simulink model "hw1_model"  (R2013a)
settings: Solver=ode45  StartTime=0.0  StopTime=10.0  RelTol=1e-3
undefined symbols (not defined in the file): c, C, k, K, m, q1_0, q1_dot_0, q2_0, q2_dot_0
settings Model: Creator=Brent  LastModifiedBy=Brent

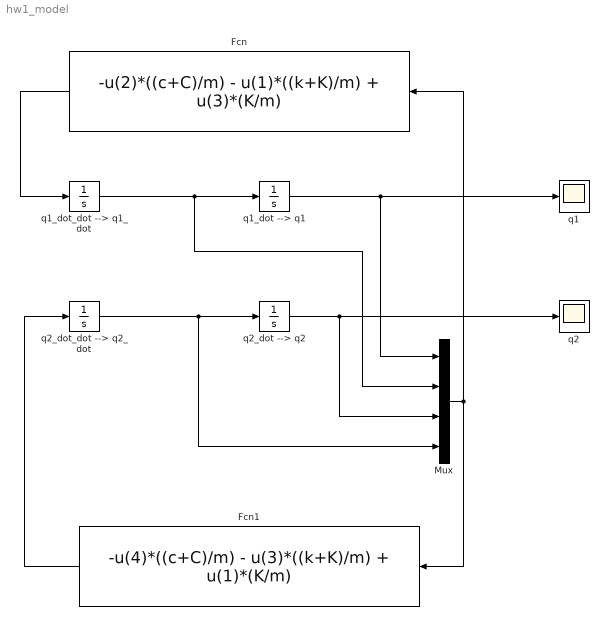
== system hw1_model ==
  Fcn : Fcn  Expr=-u(2)*((c+C)/m) - u(1)*((k+K)/m) + u(3)*(K/m)
  Fcn1 : Fcn  Expr=-u(4)*((c+C)/m) - u(3)*((k+K)/m) + u(1)*(K/m)
  Mux : Mux
  q1 : Scope
  q1_dot --> q1 : Integrator  InitialCondition=q1_0
  q1_dot_dot --> q1_dot : Integrator  InitialCondition=q1_dot_0
  q2 : Scope
  q2_dot --> q2 : Integrator  InitialCondition=q2_0
  q2_dot_dot --> q2_dot : Integrator  InitialCondition=q2_dot_0
  wires:
  q1_dot_dot --> q1_dot/1 -> q1_dot --> q1/1, Mux/2
  q2_dot_dot --> q2_dot/1 -> Mux/4, q2_dot --> q2/1
  q1_dot --> q1/1 -> Mux/1, q1/1
  q2_dot --> q2/1 -> q2/1, Mux/3
  Mux/1 -> Fcn/1, Fcn1/1
  Fcn1/1 -> q2_dot_dot --> q2_dot/1
  Fcn/1 -> q1_dot_dot --> q1_dot/1
